simulink model "test_com_SensorFusion_SF_D4_2"  (R2019b)
settings: Solver=FixedStepDiscrete  StartTime=0  StopTime=stop  FixedStep=0.001  RelTol=1e-3
undefined symbols (not defined in the file or in its folder): BxTM, ByTM, CxTM, CyTM, g, gamma_stat_front, gamma_stat_rear, gearbox_ratio, l_F, l_R, m_sprung, m_unsprung_quarter, mag_calib_front_center, mag_calib_front_compmatrix, mag_calib_rear_center, mag_calib_rear_compmatrix, should_be_in_theSensorFusion, switch_VelYcalculation_pSF, testStart_VelX_pSF, testVelY_pSF, tire_r_dyn, track_angle_front, track_width_front, track_width_rear, v2o_x, wheel_kinematics_breakpoints, wheel_kinematics_FL_data, wheel_kinematics_FR_data, wheelbase, x9DFrontX, x9DFrontY, x9DRearX, x9DRearY
libraries: SignalProcessingSensorFusionLib x30, simulink x6
(part 3 of 8)

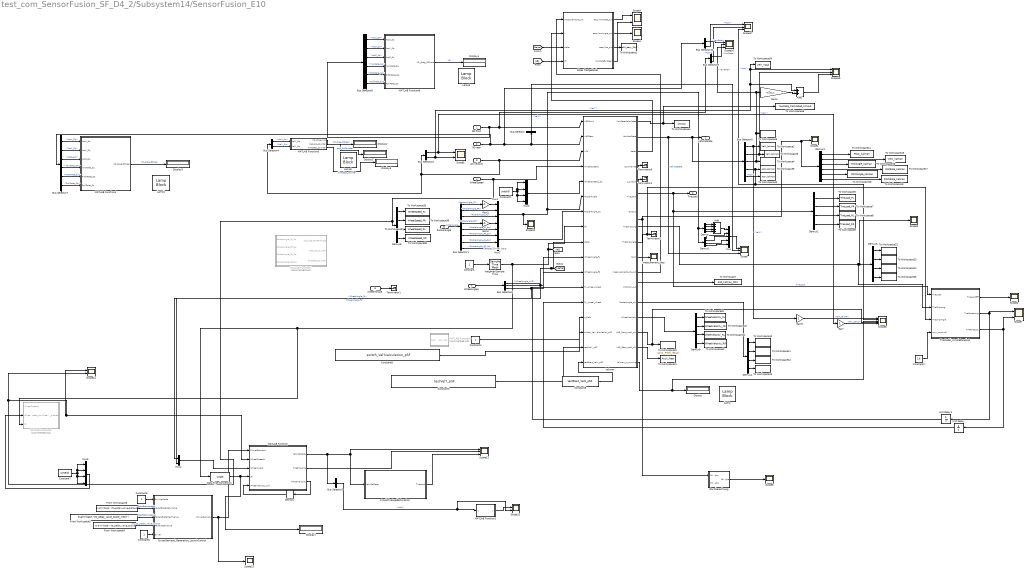
== system test_com_SensorFusion_SF_D4_2/Subsystem14/SensorFusion_E10 ==
  note: Deleted Driver Input
  9D front : Inport
  9D rear : Inport  Port=2
  v2o velocity : Inport  Port=3
  WheelSpeed : Inport  Port=4
  RockerAngle : Inport  Port=5
  WheelTorque : Inport  Port=6
  WheelAngle1 : Inport  Port=7
  Add : Sum  Inputs=++++
  Add1 : Sum
  Bus Selector : BusSelector  OutputSignals=AccX,AccY,AccZ,RollRate,PitchRate,YawRate  OutputAsBus=on
  Bus Selector1 : BusSelector  OutputSignals=RockerAngle_FL,RockerAngle_FR,RockerAngle_RL,RockerAngle_RR,RockerAngle_FL_Sq,RockerAngle_FR_Sq,RockerAngle_RL_Sq,RockerAngle_RR_Sq
  Bus Selector10 : BusSelector  OutputSignals=YawRate,AccX
  Bus Selector2 : BusSelector  OutputSignals=AccX
  Bus Selector3 : BusSelector  OutputSignals=VelX,VelY
  Bus Selector4 : BusSelector  OutputSignals=VelX_Sq,VelY_Sq
  Bus Selector5 : BusSelector  OutputSignals=VelX,VelY,YawRate,AccX,AccY
  Bus Selector6 : BusSelector  OutputSignals=WheelAngle_AVG,WheelAngle_FL,WheelAngle_FR
  Bus Selector7 : BusSelector  OutputSignals=AccX_Sq,AccY_Sq,AccZ_Sq,YawRate_Sq,PitchRate_Sq,RollRate_Sq
  Bus Selector8 : BusSelector  OutputSignals=AccX_Sq,AccY_Sq,AccZ_Sq,YawRate_Sq,PitchRate_Sq,RollRate_Sq
  Bus Selector9 : BusSelector  OutputSignals=YawRate,AccX
  Constant{,4..6} (4 alike) : Constant
  Constant1 : Constant  Value=uint8(0)
  Constant2 : Constant  Value=1.6
  Constant3 : Constant  Value=testVelY_pSF
  Constant7 : Constant  Value=uint8(0)
  Constant8 : Constant  Value=switch_VelYcalculation_pSF
  Constant9 : Constant  Value=testStart_VelX_pSF
  Data Type Conversion : DataTypeConversion  OutDataTypeStr=single
  Demux{,1..2,4..5,8..9} (7 alike) : Demux
  Demux3 : Demux  Outputs=6
  Display{,1..6} (7 alike) : Display
  DriverDemand_Generation_LaunchControl : Subsystem
  From Workspace2 : FromWorkspace  VariableName=evalin('base','VD_pedal_value_brake_mech')  SampleTime=0
  From Workspace3 : FromWorkspace  VariableName=evalin('base','VD_pedal_value_brake_rec')  SampleTime=0
  From Workspace4 : FromWorkspace  VariableName=evalin('base','VD_pedal_value_torque')  SampleTime=0
  Gain : Gain  OutDataTypeStr=single
  Gain1 : Gain  Gain=-1
  Gain2 : Gain  Gain=-1
  Gain3 : Gain  OutDataTypeStr=single
  Gain4 : Gain  Gain=-v2o_x
  Lamp{,1..3} (4 alike) : LampBlock
  MATLAB Function : MATLAB Function  TreatAsAtomicUnit=on
  MATLAB Function1 : MATLAB Function  TreatAsAtomicUnit=on
  MATLAB Function2 : MATLAB Function  Commented=on  TreatAsAtomicUnit=on
  MATLAB Function3 : MATLAB Function  Commented=on  TreatAsAtomicUnit=on
  MATLAB Function4 : MATLAB Function  TreatAsAtomicUnit=on
  MATLAB Function5 : MATLAB Function  TreatAsAtomicUnit=on
  MATLAB Function6 : MATLAB Function  TreatAsAtomicUnit=on
  MATLAB Function7 : MATLAB Function  Commented=on  TreatAsAtomicUnit=on
  Memory : Memory
  Mux : Mux  Inputs=5
  Mux{1..3,5} (4 alike) : Mux
  Mux4 : Mux  Inputs=2
  Scope{,11,15..17} (5 alike) : Scope  NumInputPorts=3
  Scope{1..2,4,6,9..10,13} (7 alike) : Scope
  Scope{3,5,7,12,14} (5 alike) : Scope  NumInputPorts=2
  Scope8 : Scope  NumInputPorts=5
  SiDes Testgelände : MATLAB Function  TreatAsAtomicUnit=on
  Sturzberechnung : Subsystem
  Terminator{1..3,6} (4 alike) : Terminator
  TireModel_simplePacejka1 : MATLAB Function  TreatAsAtomicUnit=on
  To Workspace : ToWorkspace  VariableName=e10_kalman_POS  SaveFormat=Timeseries  SampleTime=-1
  To Workspace1 : ToWorkspace  VariableName=e10_easy_POS  SaveFormat=Timeseries  SampleTime=-1
  To Workspace10 : ToWorkspace  VariableName=RockerAngle_FL  SaveFormat=Timeseries  SampleTime=-1
  To Workspace11 : ToWorkspace  VariableName=RockerAngle_FR  SaveFormat=Timeseries  SampleTime=-1
  To Workspace12 : ToWorkspace  VariableName=RockerAngle_RL  SaveFormat=Timeseries  SampleTime=-1
  To Workspace13 : ToWorkspace  VariableName=RockerAngle_RR  SaveFormat=Timeseries  SampleTime=-1
  To Workspace14 : ToWorkspace  VariableName=PosZ_kalman  SaveFormat=Timeseries  SampleTime=-1
  To Workspace15 : ToWorkspace  VariableName=VelZ_kalman  SaveFormat=Timeseries  SampleTime=-1
  To Workspace16 : ToWorkspace  VariableName=RollAngle_kalman  SaveFormat=Timeseries  SampleTime=-1
  To Workspace17 : ToWorkspace  VariableName=RollRate_kalman  SaveFormat=Timeseries  SampleTime=-1
  To Workspace18 : ToWorkspace  VariableName=PitchAngle_kalman  SaveFormat=Timeseries  SampleTime=-1
  To Workspace19 : ToWorkspace  VariableName=PitchRate_kalman  SaveFormat=Timeseries  SampleTime=-1
  To Workspace2 : ToWorkspace  VariableName=VelX_kalman  SaveFormat=Timeseries  SampleTime=-1
  To Workspace20 : ToWorkspace  VariableName=AccX_Front_result  SaveFormat=Timeseries  SampleTime=-1
  To Workspace21 : ToWorkspace  VariableName=AccX_Rear  SaveFormat=Timeseries  SampleTime=-1
  To Workspace22 : ToWorkspace  VariableName=TireSlipLong_FL  SaveFormat=Timeseries  SampleTime=-1
  To Workspace23 : ToWorkspace  VariableName=TireSlipLong_FR  SaveFormat=Timeseries  SampleTime=-1
  To Workspace24 : ToWorkspace  VariableName=TireSlipLong_RL  SaveFormat=Timeseries  SampleTime=-1
  To Workspace25 : ToWorkspace  VariableName=TireSlipLong_RR  SaveFormat=Timeseries  SampleTime=-1
  To Workspace3 : ToWorkspace  VariableName=VelY_kalman  SaveFormat=Timeseries  SampleTime=-1
  To Workspace34 : ToWorkspace  VariableName=VelY_input  SaveFormat=Timeseries  SampleTime=-1
  To Workspace35 : ToWorkspace  VariableName=WheelSpeed_FL  SaveFormat=Timeseries  SampleTime=-1
  To Workspace36 : ToWorkspace  VariableName=WheelSpeed_FR  SaveFormat=Timeseries  SampleTime=-1
  To Workspace37 : ToWorkspace  VariableName=WheelSpeed_RL  SaveFormat=Timeseries  SampleTime=-1
  To Workspace38 : ToWorkspace  VariableName=WheelSpeed_RR  SaveFormat=Timeseries  SampleTime=-1
  To Workspace39 : ToWorkspace  VariableName=WheelVelocity_FL  SaveFormat=Timeseries  SampleTime=-1
  To Workspace4 : ToWorkspace  VariableName=YawRate_kalman  SaveFormat=Timeseries  SampleTime=-1
  To Workspace40 : ToWorkspace  VariableName=WheelVelocity_FR  SaveFormat=Timeseries  SampleTime=-1
  To Workspace41 : ToWorkspace  VariableName=WheelVelocity_RL  SaveFormat=Timeseries  SampleTime=-1
  To Workspace42 : ToWorkspace  VariableName=WheelVelocity_RR  SaveFormat=Timeseries  SampleTime=-1
  To Workspace43 : ToWorkspace  VariableName=AccY_kalman  SaveFormat=Timeseries  SampleTime=-1
  To Workspace44 : ToWorkspace  VariableName=simout  SaveFormat=Timeseries  SampleTime=-1
  To Workspace45 : ToWorkspace  VariableName=YawRate_simout  SaveFormat=Timeseries  SampleTime=-1
  To Workspace46 : ToWorkspace  VariableName=YawRate_Calculated_simout  SaveFormat=Timeseries  SampleTime=-1
  To Workspace5 : ToWorkspace  VariableName=AccX_kalman  SaveFormat=Timeseries  SampleTime=-1
  To Workspace6 : ToWorkspace  VariableName=TireLoad_FL  SaveFormat=Timeseries  SampleTime=-1
  To Workspace7 : ToWorkspace  VariableName=TireLoad_FR  SaveFormat=Timeseries  SampleTime=-1
  To Workspace8 : ToWorkspace  VariableName=TireLoad_RL  SaveFormat=Timeseries  SampleTime=-1
  To Workspace9 : ToWorkspace  VariableName=TireLoad_RR  SaveFormat=Timeseries  SampleTime=-1
  Unit Delay : UnitDelay  SampleTime=-1  HasFrameUpgradeWarning=on
  Unit Delay1 : UnitDelay  SampleTime=-1  HasFrameUpgradeWarning=on
  Weighted Sample Time : SampleTimeMath  TsampMathOp=Ts Only
  kalman : MATLAB Function  TreatAsAtomicUnit=on
  measurement_bias : Scope
  simpleTireLoadEstimation : Subsystem
  VehicleState : Outport  VectorParamsAs1DForOutWhenUnconnected=off
  TireLoad : Outport  Port=2  VectorParamsAs1DForOutWhenUnconnected=off
  wires:
  Mux/1 -> Scope/1
  Demux1/4 -> Mux/5
  Demux1/3 -> Mux/4
  Demux1/2 -> Mux/3
  Demux1/1 -> Mux/2
  Add/1 -> Mux/1
  Demux/1 -> Add/1
  Demux/2 -> Add/2
  Demux/3 -> Add/3
  Demux/4 -> Add/4
  Bus Selector/1 -> Scope/2
  Gain2/1 -> Mux1/4
  Weighted Sample Time/1 -> MATLAB Function2/3(dt), Data Type Conversion/1, kalman/8(dt), [dt]
  Mux2/1 -> kalman/7(RockerAngle_Sq)
  Mux1/1 -> Scope10/1, Demux/1, Demux1/1, kalman/6(RockerAngle)
  Mux3/1 -> kalman/5(WheelSpeeds_Sq)
  Gain1/1 -> Mux1/1
  v2o velocity/1 -> Bus Selector4/1, Bus Selector3/1, kalman/3(v2o)
  9D rear/1 -> Bus Selector7/1, Bus Selector10/1, Bus Selector/1, kalman/2(x9DRear)
  Bus Selector1/5 -> Mux2/1  "<RockerAngle_FL_Sq>"
  Constant/1 -> Weighted Sample Time/1
  Constant1/1 -> Mux3/2, Mux3/1, Mux3/3, Mux3/4
  kalman/6(TireLoad) -> TireModel_simplePacejka1/1(TireLoad), Demux2/1, TireLoad/1  "TireLoad"
  Bus Selector1/7 -> Mux2/3  "<RockerAngle_RL_Sq>"
  Bus Selector1/8 -> Mux2/4  "<RockerAngle_RR_Sq>"
  Bus Selector1/3 -> Mux1/3  "<RockerAngle_RL>"
  Bus Selector1/4 -> Gain2/1  "<RockerAngle_RR>"
  WheelTorque/1 -> Terminator1/1
  RockerAngle/1 -> Bus Selector1/1  "rockerAngle"
  Bus Selector1/1 -> Gain1/1  "<RockerAngle_FL>"
  kalman/4(Covariance) -> Terminator6/1
  Bus Selector1/2 -> Mux1/2  "<RockerAngle_FR>"
  kalman/3(state) -> SiDes Testgelände/2(x)
  kalman/2(VehicleState) -> Bus Selector5/1, VehicleState/1, Scope/3  "VehicleState"
  Bus Selector1/6 -> Mux2/2  "<RockerAngle_FR_Sq>"
  kalman/12(Position_out) -> To Workspace/1
  kalman/10(bias) -> measurement_bias/1
  kalman/11(measurements_nb_out) -> SiDes Testgelände/1(measurements_nb)
  SiDes Testgelände/3(easyPos_out) -> To Workspace1/1
  SiDes Testgelände/1(easyYawRate_out) -> Scope3/1
  SiDes Testgelände/2(easyYawAngle_out) -> Scope4/1
  [dt] -> SiDes Testgelände/4(dt)
  [delta] -> SiDes Testgelände/3(delta)
  SiDes Testgelände/4(YawRateBySteer) -> Scope3/2
  Bus Selector3/1 -> Gain/1, Scope5/1  "<VelX>"
  Bus Selector3/2 -> Add1/1, Scope15/1, To Workspace34/1, Scope5/2  "<VelY>"
  Bus Selector6/2 -> Mux4/1, kalman/10(WheelAngle_FL)  "<WheelAngle_FL>"
  Bus Selector6/3 -> Mux4/2, kalman/11(WheelAngle_FR)  "<WheelAngle_FR>"
  WheelAngle1/1 -> Bus Selector6/1
  Bus Selector6/1 -> [delta], kalman/9(delta)  "<WheelAngle_AVG>"
  9D front/1 -> Bus Selector8/1, Bus Selector9/1, kalman/1(x9DFront)
  Bus Selector5/1 -> Gain3/1, To Workspace2/1  "<VelX>"
  Bus Selector5/2 -> Scope15/2, To Workspace3/1  "<VelY>"
  Bus Selector5/3 -> To Workspace45/1, Scope16/3, Gain4/1, To Workspace4/1  "<YawRate>"
  Bus Selector5/4 -> Scope17/3, Scope8/2, To Workspace5/1  "<AccX>"
  Demux2/4 -> To Workspace9/1
  Demux2/3 -> To Workspace8/1
  Demux2/2 -> To Workspace7/1
  Demux2/1 -> To Workspace6/1
  kalman/13(RockerAngle_nb) -> Demux4/1
  Demux3/1 -> To Workspace14/1
  Demux3/2 -> To Workspace15/1
  Demux3/3 -> To Workspace16/1
  Demux3/4 -> To Workspace17/1
  Demux3/5 -> To Workspace18/1
  Demux3/6 -> To Workspace19/1
  Demux4/1 -> To Workspace10/1
  Demux4/2 -> To Workspace11/1
  Demux4/3 -> To Workspace12/1
  Demux4/4 -> To Workspace13/1
  Demux5/4 -> To Workspace25/1
  Demux5/3 -> To Workspace24/1
  Demux5/2 -> To Workspace23/1
  Demux5/1 -> To Workspace22/1
  kalman/8(TireSlipLong) -> Scope9/1, Demux5/1, TireModel_simplePacejka1/2(TireSlipLong)
  Demux8/1 -> To Workspace35/1
  Demux8/2 -> To Workspace36/1
  Demux8/3 -> To Workspace37/1
  Demux8/4 -> To Workspace38/1
  Demux9/4 -> To Workspace42/1
  Demux9/3 -> To Workspace41/1
  Demux9/2 -> To Workspace40/1
  kalman/14(WheelVelocity) -> Demux9/1
  Demux9/1 -> To Workspace39/1
  Bus Selector5/5 -> To Workspace43/1  "<AccY>"
  kalman/9(TireSlipAngle) -> TireModel_simplePacejka1/3(TireSlipAngle), Terminator3/1
  kalman/5(z_output) -> Terminator2/1
  kalman/1(YawRateCalculated) -> To Workspace44/1, To Workspace46/1
  TireModel_simplePacejka1/1(TireLoadEff) -> Scope2/1
  TireModel_simplePacejka1/2(TireForceLong) -> Unit Delay1/1, Scope7/1
  Constant2/1 -> TireModel_simplePacejka1/4(mux_nominal)
  Constant4/1 -> kalman/14(c_Reib)
  TireModel_simplePacejka1/3(TireForceLat) -> Scope7/2, Unit Delay/1
  kalman/15(x9D_Front_AccX_nb) -> Scope8/4, To Workspace20/1
  kalman/16(x9D_Rear_AccX_nb) -> To Workspace21/1
  Unit Delay/1 -> kalman/13(Fy_wheel_wheel)
  Unit Delay1/1 -> kalman/12(Fx_wheel_wheel)
  kalman/7(Output) -> Sturzberechnung/1(Orientation), Demux3/1, Scope1/1
  Sturzberechnung/1(CamberAngle) -> Scope6/1
  kalman/17(kalman_is_running) -> Scope8/3, Display/1
  Gain/1 -> Scope8/5  "VelX_sensor"
  Gain3/1 -> Scope8/1  "VelX_kalman"
  simpleTireLoadEstimation/1(TireLoad) -> Scope11/3
  Memory/1 -> MATLAB Function/5(WheelVelocity_old)
  MATLAB Function/2(TireSlipLong) -> Scope11/2
  MATLAB Function/3(WheelVelocity) -> Memory/1
  Mux4/1 -> MATLAB Function/3(WheelAngle)
  DriverDemand_Generation_LaunchControl/1(DriverDemand) -> Scope13/1, MATLAB Function/1(DriverDemand)
  Constant5/1 -> DriverDemand_Generation_LaunchControl/5(Driver)
  Constant6/1 -> DriverDemand_Generation_LaunchControl/1(DrivingMode)
  From Workspace2/1 -> DriverDemand_Generation_LaunchControl/3(Pedal_BrakeMechValue)  "MechBremspedal"
  From Workspace3/1 -> DriverDemand_Generation_LaunchControl/2(PedalBrakeRecuValue)  "RekuBremspedal"
  From Workspace4/1 -> DriverDemand_Generation_LaunchControl/4(PedalAccelValue)  "ms_ad_pedal_value_torque"
  Data Type Conversion/1 -> Display1/1, MATLAB Function/4(dt)
  MATLAB Function/1(VehicleState) -> Bus Selector2/1, simpleTireLoadEstimation/1(VehicleState), Scope11/1
  Bus Selector2/1 -> Scope12/2, MATLAB Function1/1(u)  "<AccX>"
  MATLAB Function1/1(y) -> Scope12/1
  WheelSpeed/1 -> kalman/4(WheelSpeeds), MATLAB Function/2(WheelSpeeds), Scope14/1, Scope14/2, Demux8/1
  Constant7/1 -> Mux5/2, Mux5/1, Mux5/3, Mux5/4
  Mux5/1 -> MATLAB Function2/2(WheelSpeeds_Sq)
  Bus Selector4/1 -> MATLAB Function5/1(VelX_Sq)  "<VelX_Sq>"
  Bus Selector4/2 -> MATLAB Function5/2(VelY_Sq)  "<VelY_Sq>"
  MATLAB Function5/1(VD_diag_v2o) -> Display2/1  "VD_diag_9Drear"
  Bus Selector7/1 -> MATLAB Function4/1(AccX_Sq)  "<AccX_Sq>"
  Bus Selector7/2 -> MATLAB Function4/2(AccY_Sq)  "<AccY_Sq>"
  Bus Selector7/3 -> MATLAB Function4/3(AccZ_Sq)  "<AccZ_Sq>"
  Bus Selector7/4 -> MATLAB Function4/4(YawRate_Sq)  "<YawRate_Sq>"
  Bus Selector7/5 -> MATLAB Function4/5(PitchRate_Sq)  "<PitchRate_Sq>"
  Bus Selector7/6 -> MATLAB Function4/6(RollRate_Sq)  "<RollRate_Sq>"
  MATLAB Function4/1(VD_diag_9Drear) -> Display3/1  "VD_diag_9Drear"
  Bus Selector8/1 -> MATLAB Function6/1(AccX_Sq)  "<AccX_Sq>"
  Bus Selector8/2 -> MATLAB Function6/2(AccY_Sq)  "<AccY_Sq>"
  Bus Selector8/6 -> MATLAB Function6/6(RollRate_Sq)  "<RollRate_Sq>"
  Bus Selector8/5 -> MATLAB Function6/5(PitchRate_Sq)  "<PitchRate_Sq>"
  Bus Selector8/4 -> MATLAB Function6/4(YawRate_Sq)  "<YawRate_Sq>"
  Bus Selector8/3 -> MATLAB Function6/3(AccZ_Sq)  "<AccZ_Sq>"
  MATLAB Function6/1(VD_diag_9Dfront) -> Display4/1  "VD"
  MATLAB Function5/2(bad_Sq_counter) -> Display5/1  "bad_SqCounter"
  MATLAB Function5/3(timestep_counter) -> Display6/1  "timestep_counter"
  Constant8/1 -> kalman/15(switch_VelYcalculation_pSF)
  Constant3/1 -> kalman/16(testVelY_pSF)
  Gain4/1 -> Add1/2
  Add1/1 -> Scope15/3
  Bus Selector10/1 -> Scope16/1  "<YawRate>"
  Bus Selector9/1 -> Scope16/2  "<YawRate>"
  Bus Selector10/2 -> Scope17/1  "<AccX>"
  Bus Selector9/2 -> Scope17/2  "<AccX>"
  Constant9/1 -> kalman/17(testStart_VelX_pSF)

== system test_com_SensorFusion_SF_D4_2/Subsystem14/SensorFusion_E8_adjusted ==
  note: Dies ist die alte E8 Sensorfusion, die als Vergleich dient
  9D front : Inport
  9D rear : Inport  Port=2
  v2o velocity : Inport  Port=3
  WheelSpeed : Inport  Port=4  PortDimensions=4
  RockerAngle : Inport  Port=5
  WheelTorque : Inport  Port=6  PortDimensions=4
  WheelAngle : Inport  Port=7
  SensorFusion : Subsystem
  simple_TireLoadEstimation : Subsystem
  VehicleState : Outport  VectorParamsAs1DForOutWhenUnconnected=off
  TireLoad : Outport  Port=2  VectorParamsAs1DForOutWhenUnconnected=off
  wires:
  9D rear/1 -> SensorFusion/2(9D rear)
  v2o velocity/1 -> SensorFusion/3(v2o velocity)
  9D front/1 -> SensorFusion/1(9D front)
  simple_TireLoadEstimation/1(TireLoad) -> TireLoad/1  "TireLoad"
  RockerAngle/1 -> SensorFusion/5(rocker angle)
  WheelSpeed/1 -> SensorFusion/4(wheel speeds)
  WheelTorque/1 -> SensorFusion/6(wheel Torque)
  WheelAngle/1 -> SensorFusion/7(wheel Angle)
  SensorFusion/1(VehicleState) -> VehicleState/1, simple_TireLoadEstimation/1(VehicleState)  "VehicleState"

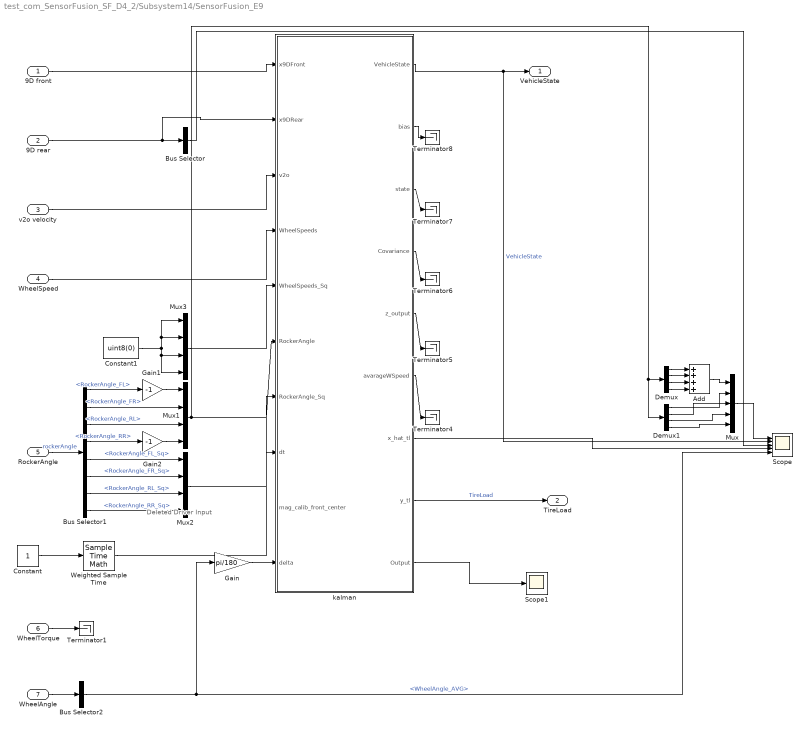
== system test_com_SensorFusion_SF_D4_2/Subsystem14/SensorFusion_E9 ==
  note: Deleted Driver Input
  9D front : Inport
  9D rear : Inport  Port=2
  v2o velocity : Inport  Port=3
  WheelSpeed : Inport  Port=4
  RockerAngle : Inport  Port=5
  WheelTorque : Inport  Port=6
  WheelAngle : Inport  Port=7
  Add : Sum  Inputs=++++
  Bus Selector : BusSelector  OutputSignals=AccX,AccY,AccZ,RollRate,PitchRate,YawRate  OutputAsBus=on
  Bus Selector1 : BusSelector  OutputSignals=RockerAngle_FL,RockerAngle_FR,RockerAngle_RL,RockerAngle_RR,RockerAngle_FL_Sq,RockerAngle_FR_Sq,RockerAngle_RL_Sq,RockerAngle_RR_Sq
  Bus Selector2 : BusSelector  OutputSignals=WheelAngle_AVG
  Constant : Constant
  Constant1 : Constant  Value=uint8(0)
  Demux : Demux
  Demux1 : Demux
  Gain : Gain  Gain=pi/180
  Gain1 : Gain  Gain=-1
  Gain2 : Gain  Gain=-1
  Mux : Mux  Inputs=5
  Mux1 : Mux
  Mux2 : Mux
  Mux3 : Mux
  Scope : Scope  NumInputPorts=5
  Scope1 : Scope
  Terminator{1,4..8} (6 alike) : Terminator
  Weighted Sample Time : SampleTimeMath  TsampMathOp=Ts Only
  kalman : MATLAB Function  TreatAsAtomicUnit=on
  VehicleState : Outport  VectorParamsAs1DForOutWhenUnconnected=off
  TireLoad : Outport  Port=2  VectorParamsAs1DForOutWhenUnconnected=off
  wires:
  Bus Selector1/6 -> Mux2/2  "<RockerAngle_FR_Sq>"
  kalman/1(VehicleState) -> Scope/2, VehicleState/1  "VehicleState"
  kalman/3(state) -> Terminator7/1
  Bus Selector1/2 -> Mux1/2  "<RockerAngle_FR>"
  kalman/4(Covariance) -> Terminator6/1
  Bus Selector1/1 -> Gain1/1  "<RockerAngle_FL>"
  RockerAngle/1 -> Bus Selector1/1  "rockerAngle"
  kalman/6(avarageWSpeed) -> Terminator4/1
  WheelTorque/1 -> Terminator1/1
  kalman/5(z_output) -> Terminator5/1
  Bus Selector1/4 -> Gain2/1  "<RockerAngle_RR>"
  kalman/2(bias) -> Terminator8/1
  WheelSpeed/1 -> kalman/4(WheelSpeeds)
  Bus Selector1/3 -> Mux1/3  "<RockerAngle_RL>"
  Bus Selector1/8 -> Mux2/4  "<RockerAngle_RR_Sq>"
  Bus Selector1/7 -> Mux2/3  "<RockerAngle_RL_Sq>"
  kalman/8(y_tl) -> TireLoad/1  "TireLoad"
  Constant1/1 -> Mux3/1, Mux3/2, Mux3/4, Mux3/3
  Constant/1 -> Weighted Sample Time/1
  Bus Selector1/5 -> Mux2/1  "<RockerAngle_FL_Sq>"
  WheelAngle/1 -> Bus Selector2/1
  9D rear/1 -> Bus Selector/1, kalman/2(x9DRear)
  v2o velocity/1 -> kalman/3(v2o)
  Gain1/1 -> Mux1/1
  9D front/1 -> kalman/1(x9DFront)
  Mux3/1 -> kalman/5(WheelSpeeds_Sq)
  Mux1/1 -> Demux1/1, Demux/1, kalman/6(RockerAngle)
  Mux2/1 -> kalman/7(RockerAngle_Sq)
  Weighted Sample Time/1 -> kalman/8(dt)
  Gain2/1 -> Mux1/4
  Bus Selector/1 -> Scope/3
  kalman/7(x_hat_tl) -> Scope/4
  Demux/4 -> Add/4
  Demux/3 -> Add/3
  Demux/2 -> Add/2
  Demux/1 -> Add/1
  Add/1 -> Mux/1
  Demux1/1 -> Mux/2
  Demux1/2 -> Mux/3
  Demux1/3 -> Mux/4
  Demux1/4 -> Mux/5
  Mux/1 -> Scope/1
  Bus Selector2/1 -> Scope/5, Gain/1  "<WheelAngle_AVG>"
  Gain/1 -> kalman/10(delta)
  kalman/9(Output) -> Scope1/1

== system test_com_SensorFusion_SF_D4_2/Subsystem14/simple_TireLoadEstimation ==
  note: Fz_FL
      | Fz_FR
      | Fz_RL
      | Fz_RR
  VehicleState : Inport  SampleTime=0.002
  Bus Selector : BusSelector  OutputSignals=AccX,AccY
  MATLAB Function : MATLAB Function  TreatAsAtomicUnit=on
  Mux2 : Mux
  TireLoad : Outport  VectorParamsAs1DForOutWhenUnconnected=off
  wires:
  Bus Selector/2 -> MATLAB Function/2(a_y)  "<AccY>"
  VehicleState/1 -> Bus Selector/1
  Bus Selector/1 -> MATLAB Function/1(a_x)  "<AccX>"
  Mux2/1 -> TireLoad/1
  MATLAB Function/1(F_z_vl) -> Mux2/1
  MATLAB Function/2(F_z_vr) -> Mux2/2
  MATLAB Function/3(F_z_hl) -> Mux2/3
  MATLAB Function/4(F_z_hr) -> Mux2/4

== system test_com_SensorFusion_SF_D4_2/Subsystem14/SensorFusion_D4/DriverDemand_Generation_LaunchControl ==
  DrivingMode : Inport
  PedalBrakeRecuValue : Inport  Port=2
  Pedal_BrakeMechValue : Inport  Port=3
  PedalAccelValue : Inport  Port=4
  Driver : Inport  Port=5
  Brake Map : Subsystem
  Logical Operator1 : Logic  Operator=NOT  AllPortsSameDT=off  OutDataTypeStr=boolean
  Memory : Memory  InheritSampleTime=on
  Rate Transition : RateTransition  OutPortSampleTime=0.01
  Rate Transition1 : RateTransition  OutPortSampleTime=0.01
  Saturation : Saturate  UpperLimit=0  LowerLimit=-1
  Saturation3 : Saturate  UpperLimit=1  LowerLimit=0
  Saturation4 : Saturate  UpperLimit=0  LowerLimit=-2
  Subsystem : Subsystem
  Subtract : Sum  Inputs=+-
  Switch : Switch  Criteria=u2 ~= 0
  Switch1 : Switch  Criteria=u2 > Threshold
  To Brake Torque : Gain  Gain=-1
  Totbereich Bremspedal : Subsystem
  Totbereich Gaspedal : Subsystem
  DriverDemand : Outport  VectorParamsAs1DForOutWhenUnconnected=off
  wires:
  Switch1/1 -> Switch/3  "Drive Request"
  Subtract/1 -> Saturation4/1  "Brake Request"
  To Brake Torque/1 -> Saturation/1
  Brake Map/1(DriverBrakeTorque) -> To Brake Torque/1
  Driver/1 -> Rate Transition/1
  Saturation/1 -> Subtract/1  "RecuBrake Request"
  Pedal_BrakeMechValue/1 -> Saturation3/1
  Saturation3/1 -> Subtract/2  "MechBrake Request"
  Saturation4/1 -> Switch/2, Switch/1
  Memory/1 -> Subsystem/3(DriverDemand_z), Switch1/3  "DriverDemand_z"
  DrivingMode/1 -> Rate Transition1/1
  Subsystem/1(AccelPedalEnable) -> Logical Operator1/1
  Totbereich Gaspedal/1(Drive Request) -> Subsystem/1(Drive Request), Switch1/1
  PedalAccelValue/1 -> Totbereich Gaspedal/1(Pedal_Accel_Value)
  PedalBrakeRecuValue/1 -> Totbereich Bremspedal/1(Pedal_BrakeRecu_Value)
  Totbereich Bremspedal/1(BrakeTorque) -> Brake Map/1(BrakeTorque)
  Logical Operator1/1 -> Switch1/2
  Rate Transition/1 -> Brake Map/2(Driver)
  Rate Transition1/1 -> Subsystem/2(DrivingMode)
  Switch/1 -> Memory/1, DriverDemand/1  "DriverDemand"

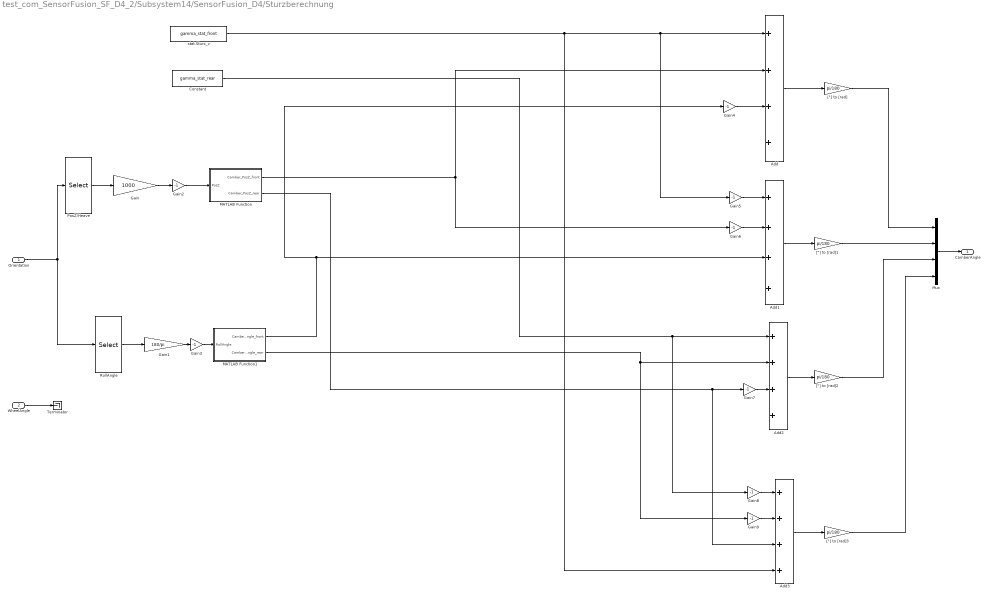
== system test_com_SensorFusion_SF_D4_2/Subsystem14/SensorFusion_D4/Sturzberechnung ==
  Orientation : Inport
  WheelAngle : Inport  Port=2
  Add{,1..3} (4 alike) : Sum  Inputs=++++
  Constant : Constant  Value=gamma_stat_rear
  Gain : Gain  Gain=1000  OutDataTypeStr=single
  Gain1 : Gain  Gain=180/pi
  Gain{2..9} (8 alike) : Gain  Gain=-1  OutDataTypeStr=single
  MATLAB Function : MATLAB Function  TreatAsAtomicUnit=on
  MATLAB Function1 : MATLAB Function  TreatAsAtomicUnit=on
  Mux : Mux
  PosZ/Heave : Selector  InputPortWidth=6  IndexOptions=Index vector (dialog)  Indices=1  OutputSizes=1
  RollAngle : Selector  InputPortWidth=6  IndexOptions=Index vector (dialog)  Indices=3  OutputSizes=1
  Terminator : Terminator
  "[°] to [rad]" : Gain  Gain=pi/180
  "[°] to [rad]1" : Gain  Gain=pi/180  OutDataTypeStr=single
  "[°] to [rad]2" : Gain  Gain=pi/180  OutDataTypeStr=single
  "[°] to [rad]3" : Gain  Gain=pi/180  OutDataTypeStr=single
  stat.Sturz_v : Constant  Value=gamma_stat_front
  CamberAngle : Outport  VectorParamsAs1DForOutWhenUnconnected=off
  wires:
  "[°] to [rad]"/1 -> Mux/1
  "[°] to [rad]1"/1 -> Mux/2
  "[°] to [rad]2"/1 -> Mux/3
  "[°] to [rad]3"/1 -> Mux/4
  Add/1 -> "[°] to [rad]"/1
  Add1/1 -> "[°] to [rad]1"/1
  Add2/1 -> "[°] to [rad]2"/1
  Add3/1 -> "[°] to [rad]3"/1
  stat.Sturz_v/1 -> Add3/4, Add/1, Gain5/1
  MATLAB Function/2(Camber_PosZ_rear) -> Add3/3, Gain7/1
  MATLAB Function1/2(Camber_RollAngle_rear) -> Gain9/1, Add2/2
  Orientation/1 -> RollAngle/1, PosZ/Heave/1
  Gain/1 -> Gain2/1
  PosZ/Heave/1 -> Gain/1
  RollAngle/1 -> Gain1/1
  Gain1/1 -> Gain3/1
  MATLAB Function1/1(Camber_RollAngle_front) -> Gain4/1, Add1/3
  Mux/1 -> CamberAngle/1
  WheelAngle/1 -> Terminator/1
  Gain2/1 -> MATLAB Function/1(PosZ)
  MATLAB Function/1(Camber_PosZ_front) -> Add/2, Gain6/1
  Constant/1 -> Add2/1, Gain8/1
  Gain3/1 -> MATLAB Function1/1(RollAngle)
  Gain4/1 -> Add/3
  Gain5/1 -> Add1/1
  Gain6/1 -> Add1/2
  Gain7/1 -> Add2/3
  Gain8/1 -> Add3/1
  Gain9/1 -> Add3/2

== system test_com_SensorFusion_SF_D4_2/Subsystem14/SensorFusion_D4/simpleTireLoadEstimation ==
  note: Fz_FL
      | Fz_FR
      | Fz_RL
      | Fz_RR
  VehicleState : Inport
  Bus Selector : BusSelector  OutputSignals=AccX,AccY
  MATLAB Function : MATLAB Function  TreatAsAtomicUnit=on
  MATLAB Function4 : MATLAB Function  TreatAsAtomicUnit=on
  Mux2 : Mux
  Scope : Scope  NumInputPorts=2
  TireLoad : Outport  VectorParamsAs1DForOutWhenUnconnected=off
  wires:
  Bus Selector/2 -> MATLAB Function/2(a_y)  "<AccY>"
  VehicleState/1 -> Bus Selector/1
  Bus Selector/1 -> Scope/1, MATLAB Function4/1(AccX)  "<AccX>"
  Mux2/1 -> TireLoad/1
  MATLAB Function/1(F_z_vl) -> Mux2/1
  MATLAB Function/2(F_z_vr) -> Mux2/2
  MATLAB Function/3(F_z_hl) -> Mux2/3
  MATLAB Function/4(F_z_hr) -> Mux2/4
  MATLAB Function4/1(AccX_out) -> Scope/2, MATLAB Function/1(a_x)

== system test_com_SensorFusion_SF_D4_2/Subsystem14/SensorFusion_E10/DriverDemand_Generation_LaunchControl ==
  DrivingMode : Inport
  PedalBrakeRecuValue : Inport  Port=2
  Pedal_BrakeMechValue : Inport  Port=3
  PedalAccelValue : Inport  Port=4
  Driver : Inport  Port=5
  Brake Map : Subsystem
  Logical Operator1 : Logic  Operator=NOT  AllPortsSameDT=off  OutDataTypeStr=boolean
  Memory : Memory  InheritSampleTime=on
  Rate Transition : RateTransition  OutPortSampleTime=0.01
  Rate Transition1 : RateTransition  OutPortSampleTime=0.01
  Saturation : Saturate  UpperLimit=0  LowerLimit=-1
  Saturation3 : Saturate  UpperLimit=1  LowerLimit=0
  Saturation4 : Saturate  UpperLimit=0  LowerLimit=-2
  Subsystem : Subsystem
  Subtract : Sum  Inputs=+-
  Switch : Switch  Criteria=u2 ~= 0
  Switch1 : Switch  Criteria=u2 > Threshold
  To Brake Torque : Gain  Gain=-1
  Totbereich Bremspedal : Subsystem
  Totbereich Gaspedal : Subsystem
  DriverDemand : Outport  VectorParamsAs1DForOutWhenUnconnected=off
  wires:
  Switch1/1 -> Switch/3  "Drive Request"
  Subtract/1 -> Saturation4/1  "Brake Request"
  To Brake Torque/1 -> Saturation/1
  Brake Map/1(DriverBrakeTorque) -> To Brake Torque/1
  Driver/1 -> Rate Transition/1
  Saturation/1 -> Subtract/1  "RecuBrake Request"
  Pedal_BrakeMechValue/1 -> Saturation3/1
  Saturation3/1 -> Subtract/2  "MechBrake Request"
  Saturation4/1 -> Switch/2, Switch/1
  Memory/1 -> Subsystem/3(DriverDemand_z), Switch1/3  "DriverDemand_z"
  DrivingMode/1 -> Rate Transition1/1
  Subsystem/1(AccelPedalEnable) -> Logical Operator1/1
  Totbereich Gaspedal/1(Drive Request) -> Subsystem/1(Drive Request), Switch1/1
  PedalAccelValue/1 -> Totbereich Gaspedal/1(Pedal_Accel_Value)
  PedalBrakeRecuValue/1 -> Totbereich Bremspedal/1(Pedal_BrakeRecu_Value)
  Totbereich Bremspedal/1(BrakeTorque) -> Brake Map/1(BrakeTorque)
  Logical Operator1/1 -> Switch1/2
  Rate Transition/1 -> Brake Map/2(Driver)
  Rate Transition1/1 -> Subsystem/2(DrivingMode)
  Switch/1 -> Memory/1, DriverDemand/1  "DriverDemand"

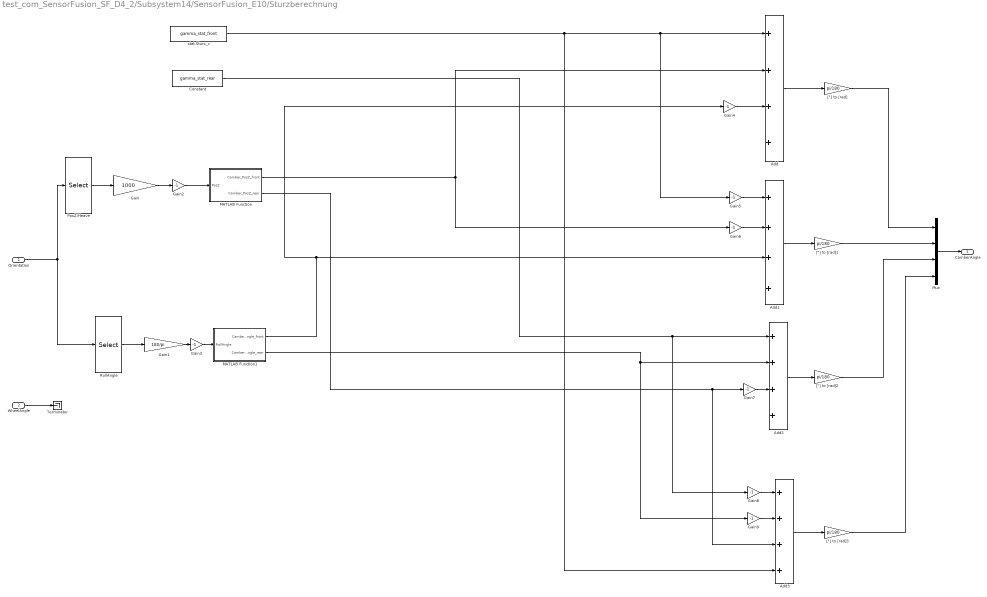
== system test_com_SensorFusion_SF_D4_2/Subsystem14/SensorFusion_E10/Sturzberechnung ==
  Orientation : Inport
  WheelAngle : Inport  Port=2
  Add{,1..3} (4 alike) : Sum  Inputs=++++
  Constant : Constant  Value=gamma_stat_rear
  Gain : Gain  Gain=1000  OutDataTypeStr=single
  Gain1 : Gain  Gain=180/pi
  Gain{2..9} (8 alike) : Gain  Gain=-1  OutDataTypeStr=single
  MATLAB Function : MATLAB Function  TreatAsAtomicUnit=on
  MATLAB Function1 : MATLAB Function  TreatAsAtomicUnit=on
  Mux : Mux
  PosZ/Heave : Selector  InputPortWidth=6  IndexOptions=Index vector (dialog)  Indices=1  OutputSizes=1
  RollAngle : Selector  InputPortWidth=6  IndexOptions=Index vector (dialog)  Indices=3  OutputSizes=1
  Terminator : Terminator
  "[°] to [rad]" : Gain  Gain=pi/180
  "[°] to [rad]1" : Gain  Gain=pi/180  OutDataTypeStr=single
  "[°] to [rad]2" : Gain  Gain=pi/180  OutDataTypeStr=single
  "[°] to [rad]3" : Gain  Gain=pi/180  OutDataTypeStr=single
  stat.Sturz_v : Constant  Value=gamma_stat_front
  CamberAngle : Outport  VectorParamsAs1DForOutWhenUnconnected=off
  wires:
  "[°] to [rad]"/1 -> Mux/1
  "[°] to [rad]1"/1 -> Mux/2
  "[°] to [rad]2"/1 -> Mux/3
  "[°] to [rad]3"/1 -> Mux/4
  Add/1 -> "[°] to [rad]"/1
  Add1/1 -> "[°] to [rad]1"/1
  Add2/1 -> "[°] to [rad]2"/1
  Add3/1 -> "[°] to [rad]3"/1
  stat.Sturz_v/1 -> Add3/4, Add/1, Gain5/1
  MATLAB Function/2(Camber_PosZ_rear) -> Add3/3, Gain7/1
  MATLAB Function1/2(Camber_RollAngle_rear) -> Gain9/1, Add2/2
  Orientation/1 -> RollAngle/1, PosZ/Heave/1
  Gain/1 -> Gain2/1
  PosZ/Heave/1 -> Gain/1
  RollAngle/1 -> Gain1/1
  Gain1/1 -> Gain3/1
  MATLAB Function1/1(Camber_RollAngle_front) -> Gain4/1, Add1/3
  Mux/1 -> CamberAngle/1
  WheelAngle/1 -> Terminator/1
  Gain2/1 -> MATLAB Function/1(PosZ)
  MATLAB Function/1(Camber_PosZ_front) -> Add/2, Gain6/1
  Constant/1 -> Add2/1, Gain8/1
  Gain3/1 -> MATLAB Function1/1(RollAngle)
  Gain4/1 -> Add/3
  Gain5/1 -> Add1/1
  Gain6/1 -> Add1/2
  Gain7/1 -> Add2/3
  Gain8/1 -> Add3/1
  Gain9/1 -> Add3/2

== system test_com_SensorFusion_SF_D4_2/Subsystem14/SensorFusion_E10/simpleTireLoadEstimation ==
  note: Fz_FL
      | Fz_FR
      | Fz_RL
      | Fz_RR
  VehicleState : Inport
  Bus Selector : BusSelector  OutputSignals=AccX,AccY
  MATLAB Function : MATLAB Function  TreatAsAtomicUnit=on
  MATLAB Function4 : MATLAB Function  TreatAsAtomicUnit=on
  Mux2 : Mux
  Scope : Scope  NumInputPorts=2
  TireLoad : Outport  VectorParamsAs1DForOutWhenUnconnected=off
  wires:
  Bus Selector/2 -> MATLAB Function/2(a_y)  "<AccY>"
  VehicleState/1 -> Bus Selector/1
  Bus Selector/1 -> Scope/1, MATLAB Function4/1(AccX)  "<AccX>"
  Mux2/1 -> TireLoad/1
  MATLAB Function/1(F_z_vl) -> Mux2/1
  MATLAB Function/2(F_z_vr) -> Mux2/2
  MATLAB Function/3(F_z_hl) -> Mux2/3
  MATLAB Function/4(F_z_hr) -> Mux2/4
  MATLAB Function4/1(AccX_out) -> Scope/2, MATLAB Function/1(a_x)

== system test_com_SensorFusion_SF_D4_2/Subsystem14/SensorFusion_E8_adjusted/SensorFusion ==
  note: DriverInput gelöscht -> bei Bedarf ChWi fragen
  9D front : Inport  SampleTime=0.002
  9D rear : Inport  Port=2  SampleTime=0.002
  v2o velocity : Inport  Port=3
  wheel speeds : Inport  Port=4
  rocker angle : Inport  Port=5
  wheel Torque : Inport  Port=6
  wheel Angle : Inport  Port=7
  Constant : Constant
  Terminator{1..4} (4 alike) : Terminator
  kalman : MATLAB Function  TreatAsAtomicUnit=on  SystemSampleTime=0.002
  VehicleState : Outport  OutDataTypeStr=Bus: control_VehicleState  VectorParamsAs1DForOutWhenUnconnected=off
  wires:
  9D rear/1 -> kalman/2(x9DRear)
  kalman/4(Covariance) -> Terminator3/1
  kalman/1(VehicleState) -> VehicleState/1
  kalman/3(Heading) -> Terminator2/1
  kalman/2(bias) -> Terminator1/1
  kalman/5(z_out) -> Terminator4/1
  9D front/1 -> kalman/1(x9DFront)
  rocker angle/1 -> kalman/5(rockerAngles)  "rockerAngle"
  Constant/1 -> kalman/8(driverInputs)
  v2o velocity/1 -> kalman/3(v2o)
  wheel speeds/1 -> kalman/4(WheelSpeeds)
  wheel Torque/1 -> kalman/6(wheelTorques)
  wheel Angle/1 -> kalman/7(wheelAngles)

== system test_com_SensorFusion_SF_D4_2/Subsystem14/SensorFusion_E8_adjusted/simple_TireLoadEstimation ==
  note: Fz_FL
      | Fz_FR
      | Fz_RL
      | Fz_RR
  VehicleState : Inport  SampleTime=0.002
  Bus Selector : BusSelector  OutputSignals=AccX,AccY
  MATLAB Function : MATLAB Function  TreatAsAtomicUnit=on
  Mux2 : Mux
  TireLoad : Outport  VectorParamsAs1DForOutWhenUnconnected=off
  wires:
  Bus Selector/2 -> MATLAB Function/2(a_y)  "<AccY>"
  VehicleState/1 -> Bus Selector/1
  Bus Selector/1 -> MATLAB Function/1(a_x)  "<AccX>"
  Mux2/1 -> TireLoad/1
  MATLAB Function/1(F_z_vl) -> Mux2/1
  MATLAB Function/2(F_z_vr) -> Mux2/2
  MATLAB Function/3(F_z_hl) -> Mux2/3
  MATLAB Function/4(F_z_hr) -> Mux2/4

== system test_com_SensorFusion_SF_D4_2/Subsystem14/SensorFusion_D4/DriverDemand_Generation_LaunchControl/Brake Map ==
  note: Bitte mit den Kennlinien unterhalb der 45 Grad Ursprungsgeraden bleiben, Einfluss auf die PowerLimitation sonst nicht auszuschließen
  note: Verschiedene Standard-Pedalmappings (ohne Geschwindigkeits- und Bremskraftfaktoreinfluss) für unterschiedliche Fahrer
  BrakeTorque : Inport
  Driver : Inport  Port=2
  AlDe : Lookup_n-D  NumberOfTableDimensions=1  BreakpointsForDimension1=[0:0.1:1]  Table=[0:0.1:1]  InternalRulePriority=Speed  RndMeth=Simplest  InputSameDT=on
  FeSch : Lookup_n-D  NumberOfTableDimensions=1  BreakpointsForDimension1=[0:0.1:1]  Table=[0:0.1:1]  InternalRulePriority=Speed  RndMeth=Simplest  InputSameDT=on
  Multiport Switch : MultiPortSwitch  DataPortOrder=Zero-based contiguous  zeroidx=on
  SiRi : Lookup_n-D  NumberOfTableDimensions=1  BreakpointsForDimension1=[0:0.1:1]  Table=[0:0.1:1]  InternalRulePriority=Speed  RndMeth=Simplest  InputSameDT=on
  DriverBrakeTorque : Outport  VectorParamsAs1DForOutWhenUnconnected=off
  wires:
  Multiport Switch/1 -> DriverBrakeTorque/1  "DriverBrakeTorque"
  BrakeTorque/1 -> AlDe/1, SiRi/1, FeSch/1
  FeSch/1 -> Multiport Switch/3
  AlDe/1 -> Multiport Switch/2
  SiRi/1 -> Multiport Switch/4
  Driver/1 -> Multiport Switch/1

== system test_com_SensorFusion_SF_D4_2/Subsystem14/SensorFusion_D4/DriverDemand_Generation_LaunchControl/Subsystem ==
  Drive Request : Inport
  DrivingMode : Inport  Port=2
  DriverDemand_z : Inport  Port=3
  "Aktiviere AccelPedalLogic nur in AccelModus " : simulink/Logic and Bit Operations/Compare To Constant  relop===  const=3  OutDataTypeStr=boolean
  EntryBedingung für AccelPedalLogic : simulink/Logic and Bit Operations/Compare To Constant  relop===  const=1  OutDataTypeStr=boolean
  LeaveBedingung für AccelPedalLogic : simulink/Logic and Bit Operations/Compare To Constant  relop=>=  const=0.5  OutDataTypeStr=boolean
  Logical Operator : Logic  Inputs=3  AllPortsSameDT=off  OutDataTypeStr=boolean
  AccelPedalEnable : Outport  VectorParamsAs1DForOutWhenUnconnected=off
  wires:
  EntryBedingung für AccelPedalLogic/1 -> Logical Operator/3
  LeaveBedingung für AccelPedalLogic/1 -> Logical Operator/1
  Logical Operator/1 -> AccelPedalEnable/1  "AccelPedalEnable"
  DrivingMode/1 -> "Aktiviere AccelPedalLogic nur in AccelModus "/1
  "Aktiviere AccelPedalLogic nur in AccelModus "/1 -> Logical Operator/2
  DriverDemand_z/1 -> EntryBedingung für AccelPedalLogic/1
  Drive Request/1 -> LeaveBedingung für AccelPedalLogic/1

== system test_com_SensorFusion_SF_D4_2/Subsystem14/SensorFusion_D4/DriverDemand_Generation_LaunchControl/Totbereich Bremspedal ==
  note: Totbereich Pedale
  Pedal_BrakeRecu_Value : Inport
  Kompensation auf ursprünglichen Wertebereich : Gain  Gain=1/0.95
  Totzone Bremspedal : DeadZone  LowerValue=0  UpperValue=0.05  SaturateOnIntegerOverflow=on
  maximaler Wert durch Totzone : Saturate  UpperLimit=0.95  LowerLimit=0
  BrakeTorque : Outport  VectorParamsAs1DForOutWhenUnconnected=off
  wires:
  maximaler Wert durch Totzone/1 -> Kompensation auf ursprünglichen Wertebereich/1
  Kompensation auf ursprünglichen Wertebereich/1 -> BrakeTorque/1  "BrakeTorque"
  Totzone Bremspedal/1 -> maximaler Wert durch Totzone/1
  Pedal_BrakeRecu_Value/1 -> Totzone Bremspedal/1  "BrakeReq"

== system test_com_SensorFusion_SF_D4_2/Subsystem14/SensorFusion_D4/DriverDemand_Generation_LaunchControl/Totbereich Gaspedal ==
  Pedal_Accel_Value : Inport
  Gain : Gain
  Kompensation auf ursprünglichen Wertebereich : Gain  Gain=1/0.98
  To Drive Torque : Gain
  Totzone Gaspedal : DeadZone  LowerValue=0  UpperValue=0.02  SaturateOnIntegerOverflow=on
  maximaler Wert durch Totzone : Saturate  UpperLimit=0.98  LowerLimit=0
  Drive Request : Outport  VectorParamsAs1DForOutWhenUnconnected=off
  wires:
  Totzone Gaspedal/1 -> maximaler Wert durch Totzone/1
  Gain/1 -> Totzone Gaspedal/1  "TorqueReq"
  maximaler Wert durch Totzone/1 -> Kompensation auf ursprünglichen Wertebereich/1
  To Drive Torque/1 -> Drive Request/1  "Drive Request"
  Pedal_Accel_Value/1 -> Gain/1
  Kompensation auf ursprünglichen Wertebereich/1 -> To Drive Torque/1

== system test_com_SensorFusion_SF_D4_2/Subsystem14/SensorFusion_E10/DriverDemand_Generation_LaunchControl/Brake Map ==
  note: Bitte mit den Kennlinien unterhalb der 45 Grad Ursprungsgeraden bleiben, Einfluss auf die PowerLimitation sonst nicht auszuschließen
  note: Verschiedene Standard-Pedalmappings (ohne Geschwindigkeits- und Bremskraftfaktoreinfluss) für unterschiedliche Fahrer
  BrakeTorque : Inport
  Driver : Inport  Port=2
  AlDe : Lookup_n-D  NumberOfTableDimensions=1  BreakpointsForDimension1=[0:0.1:1]  Table=[0:0.1:1]  InternalRulePriority=Speed  RndMeth=Simplest  InputSameDT=on
  FeSch : Lookup_n-D  NumberOfTableDimensions=1  BreakpointsForDimension1=[0:0.1:1]  Table=[0:0.1:1]  InternalRulePriority=Speed  RndMeth=Simplest  InputSameDT=on
  Multiport Switch : MultiPortSwitch  DataPortOrder=Zero-based contiguous  zeroidx=on
  SiRi : Lookup_n-D  NumberOfTableDimensions=1  BreakpointsForDimension1=[0:0.1:1]  Table=[0:0.1:1]  InternalRulePriority=Speed  RndMeth=Simplest  InputSameDT=on
  DriverBrakeTorque : Outport  VectorParamsAs1DForOutWhenUnconnected=off
  wires:
  Multiport Switch/1 -> DriverBrakeTorque/1  "DriverBrakeTorque"
  BrakeTorque/1 -> AlDe/1, SiRi/1, FeSch/1
  FeSch/1 -> Multiport Switch/3
  AlDe/1 -> Multiport Switch/2
  SiRi/1 -> Multiport Switch/4
  Driver/1 -> Multiport Switch/1

== system test_com_SensorFusion_SF_D4_2/Subsystem14/SensorFusion_E10/DriverDemand_Generation_LaunchControl/Subsystem ==
  Drive Request : Inport
  DrivingMode : Inport  Port=2
  DriverDemand_z : Inport  Port=3
  "Aktiviere AccelPedalLogic nur in AccelModus " : simulink/Logic and Bit Operations/Compare To Constant  relop===  const=3  OutDataTypeStr=boolean
  EntryBedingung für AccelPedalLogic : simulink/Logic and Bit Operations/Compare To Constant  relop===  const=1  OutDataTypeStr=boolean
  LeaveBedingung für AccelPedalLogic : simulink/Logic and Bit Operations/Compare To Constant  relop=>=  const=0.5  OutDataTypeStr=boolean
  Logical Operator : Logic  Inputs=3  AllPortsSameDT=off  OutDataTypeStr=boolean
  AccelPedalEnable : Outport  VectorParamsAs1DForOutWhenUnconnected=off
  wires:
  EntryBedingung für AccelPedalLogic/1 -> Logical Operator/3
  LeaveBedingung für AccelPedalLogic/1 -> Logical Operator/1
  Logical Operator/1 -> AccelPedalEnable/1  "AccelPedalEnable"
  DrivingMode/1 -> "Aktiviere AccelPedalLogic nur in AccelModus "/1
  "Aktiviere AccelPedalLogic nur in AccelModus "/1 -> Logical Operator/2
  DriverDemand_z/1 -> EntryBedingung für AccelPedalLogic/1
  Drive Request/1 -> LeaveBedingung für AccelPedalLogic/1

== system test_com_SensorFusion_SF_D4_2/Subsystem14/SensorFusion_E10/DriverDemand_Generation_LaunchControl/Totbereich Bremspedal ==
  note: Totbereich Pedale
  Pedal_BrakeRecu_Value : Inport
  Kompensation auf ursprünglichen Wertebereich : Gain  Gain=1/0.95
  Totzone Bremspedal : DeadZone  LowerValue=0  UpperValue=0.05  SaturateOnIntegerOverflow=on
  maximaler Wert durch Totzone : Saturate  UpperLimit=0.95  LowerLimit=0
  BrakeTorque : Outport  VectorParamsAs1DForOutWhenUnconnected=off
  wires:
  maximaler Wert durch Totzone/1 -> Kompensation auf ursprünglichen Wertebereich/1
  Kompensation auf ursprünglichen Wertebereich/1 -> BrakeTorque/1  "BrakeTorque"
  Totzone Bremspedal/1 -> maximaler Wert durch Totzone/1
  Pedal_BrakeRecu_Value/1 -> Totzone Bremspedal/1  "BrakeReq"

== system test_com_SensorFusion_SF_D4_2/Subsystem14/SensorFusion_E10/DriverDemand_Generation_LaunchControl/Totbereich Gaspedal ==
  Pedal_Accel_Value : Inport
  Gain : Gain
  Kompensation auf ursprünglichen Wertebereich : Gain  Gain=1/0.98
  To Drive Torque : Gain
  Totzone Gaspedal : DeadZone  LowerValue=0  UpperValue=0.02  SaturateOnIntegerOverflow=on
  maximaler Wert durch Totzone : Saturate  UpperLimit=0.98  LowerLimit=0
  Drive Request : Outport  VectorParamsAs1DForOutWhenUnconnected=off
  wires:
  Totzone Gaspedal/1 -> maximaler Wert durch Totzone/1
  Gain/1 -> Totzone Gaspedal/1  "TorqueReq"
  maximaler Wert durch Totzone/1 -> Kompensation auf ursprünglichen Wertebereich/1
  To Drive Torque/1 -> Drive Request/1  "Drive Request"
  Pedal_Accel_Value/1 -> Gain/1
  Kompensation auf ursprünglichen Wertebereich/1 -> To Drive Torque/1
